simulink model "Lab10_questao_01_plantas"  (Simulink 6.6)
settings: Solver=ode45  StartTime=0.0  StopTime=5  RelTol=1e-3
InitFcn:
  | A = [1 1 0;-12 0 1;20 0 0];
  | 
  | B1 = [0;1;1];
  | 
  | C = [21 -1 1;1 0 0 ;0 1 0;0 0 1];
  | 
  | D=[0; 0; 0; 0];
settings Model: Creator=ALUNO  LastModifiedBy=Rawlinson
settings GRTTargetCC: TargetFcnLib=ansi_tfl_table_tmw.mat

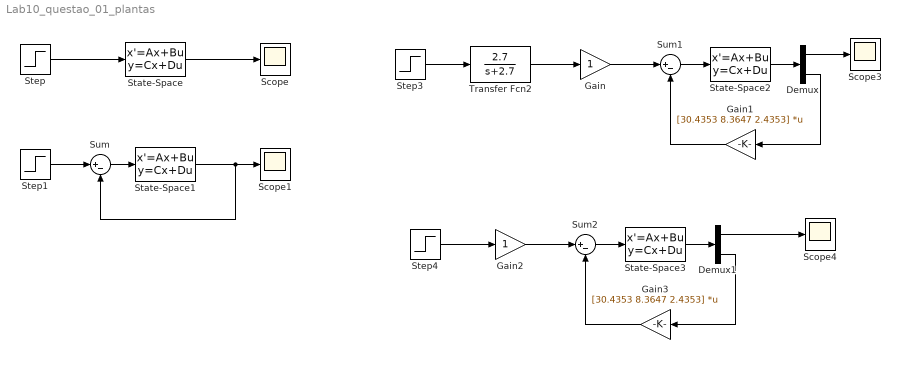
== system Lab10_questao_01_plantas ==
  Demux : Demux  Outputs=[1 3]
  Demux1 : Demux  Outputs=[1 3]
  Gain : Gain
  Gain1 : Gain  Orientation=left  Gain=[30.4353 8.3647 2.4353]  Multiplication=Matrix(K*u) (u vector)
  Gain2 : Gain
  Gain3 : Gain  Orientation=left  Gain=[30.4353 8.3647 2.4353]  Multiplication=Matrix(K*u) (u vector)
  Scope{,1,3..4} (4 alike) : Scope
      Scope1 settings: TimeRange=5  YMin=-20  YMax=40
      Scope3 settings: TimeRange=100  YMin=0  YMax=1.2e+068  SaveName=ScopeData3
      Scope4 settings: TimeRange=100  YMin=0  YMax=1.2e+068  SaveName=ScopeData4
  State-Space : StateSpace  A=[1 1 0; -12 0 1; 20 0 0]  B=[0; 1; 1]  C=[21 -1 1]  D=[0]
  State-Space1 : StateSpace  A=[1 1 0; -12 0 1; 20 0 0]  B=[0; 1; 1]  C=[21 -1 1]  D=[0]
  State-Space2 : StateSpace  A=A  B=B1  C=C  D=D
  State-Space3 : StateSpace  A=A  B=B1  C=C  D=D
  Step : Step  SampleTime=0
  Step1 : Step  SampleTime=0
  Step3 : Step  Time=0  SampleTime=0
  Step4 : Step  Time=0  SampleTime=0
  Sum : Sum  Inputs=|+-
  Sum1 : Sum  Inputs=|+-
  Sum2 : Sum  Inputs=|+-
  Transfer Fcn2 : TransferFcn  InitFcn=|  Numerator=[2.7]  Denominator=[1 2.7]
      | J=0.5;
      | B=0;  
      | O=10; 
      | r=1;  
      | R=49; 
      | K=4;  
      | E=9;
  wires:
  Step/1 -> State-Space/1
  State-Space/1 -> Scope/1
  State-Space1/1 -> Scope1/1, Sum/2
  Sum/1 -> State-Space1/1
  Step1/1 -> Sum/1
  State-Space2/1 -> Demux/1
  Sum1/1 -> State-Space2/1
  Gain1/1 -> Sum1/2
  Demux/2 -> Gain1/1
  Transfer Fcn2/1 -> Gain/1
  Demux/1 -> Scope3/1
  Gain/1 -> Sum1/1
  Step3/1 -> Transfer Fcn2/1
  State-Space3/1 -> Demux1/1
  Sum2/1 -> State-Space3/1
  Gain3/1 -> Sum2/2
  Demux1/2 -> Gain3/1
  Demux1/1 -> Scope4/1
  Gain2/1 -> Sum2/1
  Step4/1 -> Gain2/1
